simulink model "Thirtybussys_final"  (R2023b)
settings: Solver=VariableStepAuto  StartTime=0.0  StopTime=0.7  RelTol=1e-3
libraries: eePowerMeasurement x60, spsFourierLib x60, spsThreePhaseSeriesRLCBranchLib x41, spsThreePhaseVIMeasurementLib x30, spsThreePhaseSeriesRLCLoadLib x21, spsThreePhaseSourceLib x6, spsThreePhaseTransformerTwoWindingsLib x6, spsThreePhaseFaultLib x2, spspowerguiLib x1
(part 3 of 3)

== system Thirtybussys_final/Voltage /Per Unit Voltage19 ==
  In1 : Inport
  Demux : Demux  Outputs=3
  Fourier : spsFourierLib/Fourier  Freq=60  n=1  InInit=[0, 0]  Ts=50e-6
  Gain : Gain  Gain=1/3
  Sum : Sum  Inputs=|+++
  Out1 : Outport  VectorParamsAs1DForOutWhenUnconnected=off
  wires:
  In1/1 -> Fourier/1
  Gain/1 -> Out1/1
  Fourier/1 -> Demux/1
  Demux/1 -> Sum/1
  Demux/2 -> Sum/2
  Demux/3 -> Sum/3
  Sum/1 -> Gain/1

== system Thirtybussys_final/Voltage /Per Unit Voltage2 ==
  In1 : Inport
  Demux : Demux  Outputs=3
  Fourier : spsFourierLib/Fourier  Freq=60  n=1  InInit=[0, 0]  Ts=50e-6
  Gain : Gain  Gain=1/3
  Sum : Sum  Inputs=|+++
  Out1 : Outport  VectorParamsAs1DForOutWhenUnconnected=off
  wires:
  In1/1 -> Fourier/1
  Gain/1 -> Out1/1
  Fourier/1 -> Demux/1
  Demux/1 -> Sum/1
  Demux/2 -> Sum/2
  Demux/3 -> Sum/3
  Sum/1 -> Gain/1

== system Thirtybussys_final/Voltage /Per Unit Voltage20 ==
  In1 : Inport
  Demux : Demux  Outputs=3
  Fourier : spsFourierLib/Fourier  Freq=60  n=1  InInit=[0, 0]  Ts=50e-6
  Gain : Gain  Gain=1/3
  Sum : Sum  Inputs=|+++
  Out1 : Outport  VectorParamsAs1DForOutWhenUnconnected=off
  wires:
  Sum/1 -> Gain/1
  Demux/3 -> Sum/3
  Demux/2 -> Sum/2
  Demux/1 -> Sum/1
  Fourier/1 -> Demux/1
  Gain/1 -> Out1/1
  In1/1 -> Fourier/1

== system Thirtybussys_final/Voltage /Per Unit Voltage21 ==
  In1 : Inport
  Demux : Demux  Outputs=3
  Fourier : spsFourierLib/Fourier  Freq=60  n=1  InInit=[0, 0]  Ts=50e-6
  Gain : Gain  Gain=1/3
  Sum : Sum  Inputs=|+++
  Out1 : Outport  VectorParamsAs1DForOutWhenUnconnected=off
  wires:
  In1/1 -> Fourier/1
  Gain/1 -> Out1/1
  Fourier/1 -> Demux/1
  Demux/1 -> Sum/1
  Demux/2 -> Sum/2
  Demux/3 -> Sum/3
  Sum/1 -> Gain/1

== system Thirtybussys_final/Voltage /Per Unit Voltage22 ==
  In1 : Inport
  Demux : Demux  Outputs=3
  Fourier : spsFourierLib/Fourier  Freq=60  n=1  InInit=[0, 0]  Ts=50e-6
  Gain : Gain  Gain=1/3
  Sum : Sum  Inputs=|+++
  Out1 : Outport  VectorParamsAs1DForOutWhenUnconnected=off
  wires:
  Sum/1 -> Gain/1
  Demux/3 -> Sum/3
  Demux/2 -> Sum/2
  Demux/1 -> Sum/1
  Fourier/1 -> Demux/1
  Gain/1 -> Out1/1
  In1/1 -> Fourier/1

== system Thirtybussys_final/Voltage /Per Unit Voltage23 ==
  In1 : Inport
  Demux : Demux  Outputs=3
  Fourier : spsFourierLib/Fourier  Freq=60  n=1  InInit=[0, 0]  Ts=50e-6
  Gain : Gain  Gain=1/3
  Sum : Sum  Inputs=|+++
  Out1 : Outport  VectorParamsAs1DForOutWhenUnconnected=off
  wires:
  In1/1 -> Fourier/1
  Gain/1 -> Out1/1
  Fourier/1 -> Demux/1
  Demux/1 -> Sum/1
  Demux/2 -> Sum/2
  Demux/3 -> Sum/3
  Sum/1 -> Gain/1

== system Thirtybussys_final/Voltage /Per Unit Voltage24 ==
  In1 : Inport
  Demux : Demux  Outputs=3
  Fourier : spsFourierLib/Fourier  Freq=60  n=1  InInit=[0, 0]  Ts=50e-6
  Gain : Gain  Gain=1/3
  Sum : Sum  Inputs=|+++
  Out1 : Outport  VectorParamsAs1DForOutWhenUnconnected=off
  wires:
  In1/1 -> Fourier/1
  Gain/1 -> Out1/1
  Fourier/1 -> Demux/1
  Demux/1 -> Sum/1
  Demux/2 -> Sum/2
  Demux/3 -> Sum/3
  Sum/1 -> Gain/1

== system Thirtybussys_final/Voltage /Per Unit Voltage25 ==
  In1 : Inport
  Demux : Demux  Outputs=3
  Fourier : spsFourierLib/Fourier  Freq=60  n=1  InInit=[0, 0]  Ts=50e-6
  Gain : Gain  Gain=1/3
  Sum : Sum  Inputs=|+++
  Out1 : Outport  VectorParamsAs1DForOutWhenUnconnected=off
  wires:
  Sum/1 -> Gain/1
  Demux/3 -> Sum/3
  Demux/2 -> Sum/2
  Demux/1 -> Sum/1
  Fourier/1 -> Demux/1
  Gain/1 -> Out1/1
  In1/1 -> Fourier/1

== system Thirtybussys_final/Voltage /Per Unit Voltage26 ==
  In1 : Inport
  Demux : Demux  Outputs=3
  Fourier : spsFourierLib/Fourier  Freq=60  n=1  InInit=[0, 0]  Ts=50e-6
  Gain : Gain  Gain=1/3
  Sum : Sum  Inputs=|+++
  Out1 : Outport  VectorParamsAs1DForOutWhenUnconnected=off
  wires:
  In1/1 -> Fourier/1
  Gain/1 -> Out1/1
  Fourier/1 -> Demux/1
  Demux/1 -> Sum/1
  Demux/2 -> Sum/2
  Demux/3 -> Sum/3
  Sum/1 -> Gain/1

== system Thirtybussys_final/Voltage /Per Unit Voltage27 ==
  In1 : Inport
  Demux : Demux  Outputs=3
  Fourier : spsFourierLib/Fourier  Freq=60  n=1  InInit=[0, 0]  Ts=50e-6
  Gain : Gain  Gain=1/3
  Sum : Sum  Inputs=|+++
  Out1 : Outport  VectorParamsAs1DForOutWhenUnconnected=off
  wires:
  Sum/1 -> Gain/1
  Demux/3 -> Sum/3
  Demux/2 -> Sum/2
  Demux/1 -> Sum/1
  Fourier/1 -> Demux/1
  Gain/1 -> Out1/1
  In1/1 -> Fourier/1

== system Thirtybussys_final/Voltage /Per Unit Voltage28 ==
  In1 : Inport
  Demux : Demux  Outputs=3
  Fourier : spsFourierLib/Fourier  Freq=60  n=1  InInit=[0, 0]  Ts=50e-6
  Gain : Gain  Gain=1/3
  Sum : Sum  Inputs=|+++
  Out1 : Outport  VectorParamsAs1DForOutWhenUnconnected=off
  wires:
  In1/1 -> Fourier/1
  Gain/1 -> Out1/1
  Fourier/1 -> Demux/1
  Demux/1 -> Sum/1
  Demux/2 -> Sum/2
  Demux/3 -> Sum/3
  Sum/1 -> Gain/1

== system Thirtybussys_final/Voltage /Per Unit Voltage29 ==
  In1 : Inport
  Demux : Demux  Outputs=3
  Fourier : spsFourierLib/Fourier  Freq=60  n=1  InInit=[0, 0]  Ts=50e-6
  Gain : Gain  Gain=1/3
  Sum : Sum  Inputs=|+++
  Out1 : Outport  VectorParamsAs1DForOutWhenUnconnected=off
  wires:
  Sum/1 -> Gain/1
  Demux/3 -> Sum/3
  Demux/2 -> Sum/2
  Demux/1 -> Sum/1
  Fourier/1 -> Demux/1
  Gain/1 -> Out1/1
  In1/1 -> Fourier/1

== system Thirtybussys_final/Voltage /Per Unit Voltage3 ==
  In1 : Inport
  Demux : Demux  Outputs=3
  Fourier : spsFourierLib/Fourier  Freq=60  n=1  InInit=[0, 0]  Ts=50e-6
  Gain : Gain  Gain=1/3
  Sum : Sum  Inputs=|+++
  Out1 : Outport  VectorParamsAs1DForOutWhenUnconnected=off
  wires:
  Sum/1 -> Gain/1
  Demux/3 -> Sum/3
  Demux/2 -> Sum/2
  Demux/1 -> Sum/1
  Fourier/1 -> Demux/1
  Gain/1 -> Out1/1
  In1/1 -> Fourier/1

== system Thirtybussys_final/Voltage /Per Unit Voltage4 ==
  In1 : Inport
  Demux : Demux  Outputs=3
  Fourier : spsFourierLib/Fourier  Freq=60  n=1  InInit=[0, 0]  Ts=50e-6
  Gain : Gain  Gain=1/3
  Sum : Sum  Inputs=|+++
  Out1 : Outport  VectorParamsAs1DForOutWhenUnconnected=off
  wires:
  In1/1 -> Fourier/1
  Gain/1 -> Out1/1
  Fourier/1 -> Demux/1
  Demux/1 -> Sum/1
  Demux/2 -> Sum/2
  Demux/3 -> Sum/3
  Sum/1 -> Gain/1

== system Thirtybussys_final/Voltage /Per Unit Voltage5 ==
  In1 : Inport
  Demux : Demux  Outputs=3
  Fourier : spsFourierLib/Fourier  Freq=60  n=1  InInit=[0, 0]  Ts=50e-6
  Gain : Gain  Gain=1/3
  Sum : Sum  Inputs=|+++
  Out1 : Outport  VectorParamsAs1DForOutWhenUnconnected=off
  wires:
  Sum/1 -> Gain/1
  Demux/3 -> Sum/3
  Demux/2 -> Sum/2
  Demux/1 -> Sum/1
  Fourier/1 -> Demux/1
  Gain/1 -> Out1/1
  In1/1 -> Fourier/1

== system Thirtybussys_final/Voltage /Per Unit Voltage6 ==
  In1 : Inport
  Demux : Demux  Outputs=3
  Fourier : spsFourierLib/Fourier  Freq=60  n=1  InInit=[0, 0]  Ts=50e-6
  Gain : Gain  Gain=1/3
  Sum : Sum  Inputs=|+++
  Out1 : Outport  VectorParamsAs1DForOutWhenUnconnected=off
  wires:
  Sum/1 -> Gain/1
  Demux/3 -> Sum/3
  Demux/2 -> Sum/2
  Demux/1 -> Sum/1
  Fourier/1 -> Demux/1
  Gain/1 -> Out1/1
  In1/1 -> Fourier/1

== system Thirtybussys_final/Voltage /Per Unit Voltage7 ==
  In1 : Inport
  Demux : Demux  Outputs=3
  Fourier : spsFourierLib/Fourier  Freq=60  n=1  InInit=[0, 0]  Ts=50e-6
  Gain : Gain  Gain=1/3
  Sum : Sum  Inputs=|+++
  Out1 : Outport  VectorParamsAs1DForOutWhenUnconnected=off
  wires:
  In1/1 -> Fourier/1
  Gain/1 -> Out1/1
  Fourier/1 -> Demux/1
  Demux/1 -> Sum/1
  Demux/2 -> Sum/2
  Demux/3 -> Sum/3
  Sum/1 -> Gain/1

== system Thirtybussys_final/Voltage /Per Unit Voltage8 ==
  In1 : Inport
  Demux : Demux  Outputs=3
  Fourier : spsFourierLib/Fourier  Freq=60  n=1  InInit=[0, 0]  Ts=50e-6
  Gain : Gain  Gain=1/3
  Sum : Sum  Inputs=|+++
  Out1 : Outport  VectorParamsAs1DForOutWhenUnconnected=off
  wires:
  Sum/1 -> Gain/1
  Demux/3 -> Sum/3
  Demux/2 -> Sum/2
  Demux/1 -> Sum/1
  Fourier/1 -> Demux/1
  Gain/1 -> Out1/1
  In1/1 -> Fourier/1

== system Thirtybussys_final/Voltage /Per Unit Voltage9 ==
  In1 : Inport
  Demux : Demux  Outputs=3
  Fourier : spsFourierLib/Fourier  Freq=60  n=1  InInit=[0, 0]  Ts=50e-6
  Gain : Gain  Gain=1/3
  Sum : Sum  Inputs=|+++
  Out1 : Outport  VectorParamsAs1DForOutWhenUnconnected=off
  wires:
  In1/1 -> Fourier/1
  Gain/1 -> Out1/1
  Fourier/1 -> Demux/1
  Demux/1 -> Sum/1
  Demux/2 -> Sum/2
  Demux/3 -> Sum/3
  Sum/1 -> Gain/1
